simulink model "Test"  (R2024b)
settings: Solver=FixedStepAuto  StartTime=0.0  StopTime=20  FixedStep=0.001  RelTol=1e-3
libraries: simulink x1, fuzblock x1
settings Model: Creator=Liu Sha  LastModifiedBy=Liu Sha

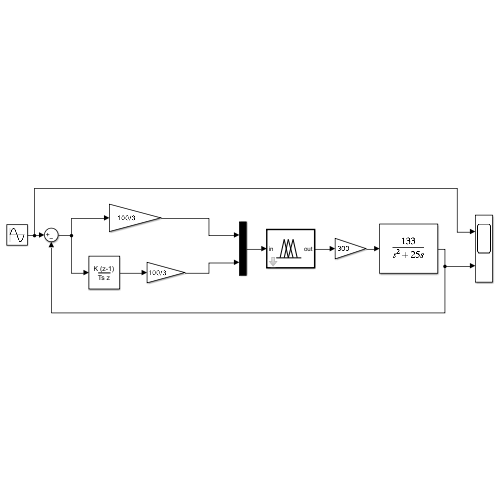
[thumbnail: Simulink's stored preview of the top-level diagram]
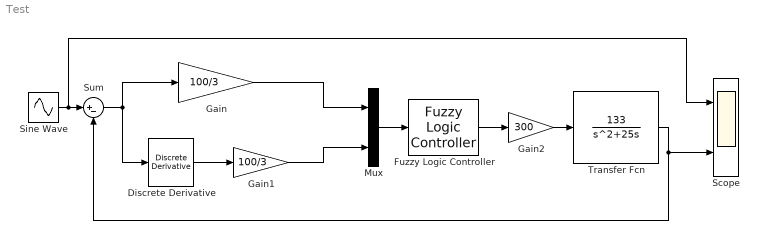
== system Test ==
  Discrete Derivative : simulink/Discrete/Discrete Derivative  gainval=1.0  ICPrevScaledInput=0.0  OutMin=[]  OutMax=[]  OutDataType=fixdt(1, 16)  OutScaling=2^-10  DoSatur=off
  Fuzzy Logic Controller : fuzblock/Fuzzy Logic  Controller  FIS='Test.fis'  OutputSampleNumber=101  DataType=double  FuzzifiedInputs=off  RuleFiringStrengths=off  RuleOutputs=off  AggregatedOutputs=off  SimulateUsing=Interpreted execution  OutOfRangeInputValueMessage=warning  NoRuleFiredMessage=warning  EmptyOutputFuzzySetMessage=warning
  Gain : Gain  Gain=100/3
  Gain1 : Gain  Gain=100/3
  Gain2 : Gain  Gain=300
  Mux : Mux  Inputs=2
  Scope : Scope  NumInputPorts=2
  Sine Wave : Sin  Frequency=10  SampleTime=0
  Sum : Sum  Inputs=|+-
  Transfer Fcn : TransferFcn  Numerator=[133]  Denominator=[1 25 0]
  wires:
  Sum/1 -> Discrete Derivative/1, Gain/1
  Sine Wave/1 -> Scope/1, Sum/1
  Discrete Derivative/1 -> Gain1/1
  Fuzzy Logic Controller/1 -> Gain2/1
  Gain2/1 -> Transfer Fcn/1
  Transfer Fcn/1 -> Sum/2, Scope/2
  Gain/1 -> Mux/1
  Mux/1 -> Fuzzy Logic Controller/1
  Gain1/1 -> Mux/2
